simulink model "MPCController"  (R2024a)
settings: configuration reference "csMultiInstance" (kept outside this file)
undefined symbols (not defined in the file or in its folder): longVelLlimit, longVelUlimit, mioIgnoreDistanceThreshold, mioIgnoreRelDistance, mioIgnoreVelocity, time_gap, Ts
libraries: mpcadaslib x1
Description:
  | Model Predictive Controller Model. This is considered as a SW unit.
settings Model: DataDictionary=DD_MPCController.sldd  EnableAccessToBaseWorkspace=off  Creator=The MathWorks, Inc.  LastModifiedBy=The MathWorks, Inc.
settings ConfigSetRef: SourceName=csMultiInstance

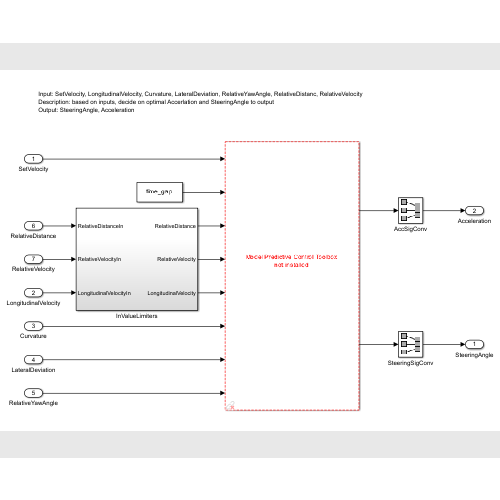
[thumbnail: Simulink's stored preview of the top-level diagram]
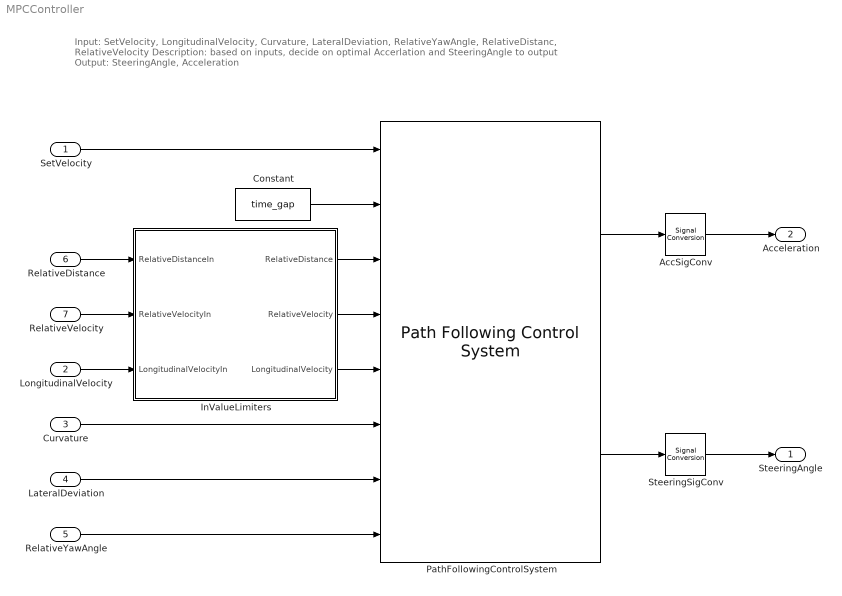
== system MPCController ==
  note: Input: SetVelocity, LongitudinalVelocity, Curvature, LateralDeviation, RelativeYawAngle, RelativeDistanc, RelativeVelocity
      | Description: based on inputs, decide on optimal Accerlation and SteeringAngle to output
      | Output: SteeringAngle, Acceleration
  SetVelocity : Inport  OutMin=-realmax  OutMax=realmax  OutDataTypeStr=double  Unit=m/s  PortDimensions=1  SampleTime=Ts
  LongitudinalVelocity : Inport  Port=2  OutMin=-realmax  OutMax=realmax  OutDataTypeStr=double  Unit=m/s  PortDimensions=1  SampleTime=Ts
  Curvature : Inport  Port=3  OutMin=-realmax  OutMax=realmax  OutDataTypeStr=double  PortDimensions=PredictionNumSteps  SampleTime=Ts
  LateralDeviation : Inport  Port=4  OutMin=-realmax  OutMax=realmax  OutDataTypeStr=double  PortDimensions=1  SampleTime=Ts
  RelativeYawAngle : Inport  Port=5  OutMin=-realmax  OutMax=realmax  OutDataTypeStr=double  Unit=rad  PortDimensions=1  SampleTime=Ts
  RelativeDistance : Inport  Port=6  OutMin=-realmax  OutMax=realmax  OutDataTypeStr=double  Unit=m  PortDimensions=1  SampleTime=Ts
  RelativeVelocity : Inport  Port=7  OutMin=-realmax  OutMax=realmax  OutDataTypeStr=double  Unit=m/s  PortDimensions=1  SampleTime=Ts
  AccSigConv : SignalConversion  OverrideOpt=off
  Constant : Constant  Value=time_gap
  InValueLimiters : Subsystem
  PathFollowingControlSystem : mpcadaslib/Path Following Control System  VariantControl=Variant2  ModelType=Use vehicle parameters  VehicleMass=m  VehicleYawInertia=Iz  LengthToFront=lf  LengthToRear=lr  FrontTireStiffness=Cf  RearTireStiffness=Cr  AccelTimeConstant=tau  EgoModelMatrixA=[-2,zeros(1,3);1,zeros(1,3);zeros(1,2),-4.4021,-12.4603;zeros(1,2),1.3913,-5.1868]  EgoModelMatrixB=[2,zeros(1,3);zeros(1,2),24.1270,15.8609]'  EgoModelMatrixC=[zeros(3,1),eye(3)]  InitialLongVel=v0_ego  TransportLag=Ts  spaceCtrl=on  DefaultSpacing=default_spacing  MinSteering=min_steer  umin_ext=off  MaxSteering=max_steer  umax_ext=off  MinAcceleration=min_ac  amin_ext=off  MaxAcceleration=max_ac  amax_ext=off  Ts=Ts  PredictionHorizon=30  ControlHorizon=3  LongWeight=0.1  LateralWeight=1  AccelRateWeight=0.1  SteerRateWeight=0.1  suboptimal=off  maxiter=10  datatypeopt=double  optmode=off  trackmode=off
  SteeringSigConv : SignalConversion  OverrideOpt=off
  SteeringAngle : Outport  OutMin=-realmax  OutMax=realmax  OutDataTypeStr=double  Unit=rad  PortDimensions=1  SampleTime=Ts  VectorParamsAs1DForOutWhenUnconnected=off
  Acceleration : Outport  Port=2  OutMin=-realmax  OutMax=realmax  OutDataTypeStr=double  Unit=m/s^2  PortDimensions=1  SampleTime=Ts  VectorParamsAs1DForOutWhenUnconnected=off
  wires:
  RelativeYawAngle/1 -> PathFollowingControlSystem/8
  PathFollowingControlSystem/1 -> AccSigConv/1
  PathFollowingControlSystem/2 -> SteeringSigConv/1
  LateralDeviation/1 -> PathFollowingControlSystem/7
  Curvature/1 -> PathFollowingControlSystem/6
  SetVelocity/1 -> PathFollowingControlSystem/1
  Constant/1 -> PathFollowingControlSystem/2
  RelativeDistance/1 -> InValueLimiters/1(RelativeDistanceIn)
  RelativeVelocity/1 -> InValueLimiters/2(RelativeVelocityIn)
  LongitudinalVelocity/1 -> InValueLimiters/3(LongitudinalVelocityIn)
  InValueLimiters/1(RelativeDistance) -> PathFollowingControlSystem/3
  InValueLimiters/2(RelativeVelocity) -> PathFollowingControlSystem/4
  InValueLimiters/3(LongitudinalVelocity) -> PathFollowingControlSystem/5
  SteeringSigConv/1 -> SteeringAngle/1
  AccSigConv/1 -> Acceleration/1

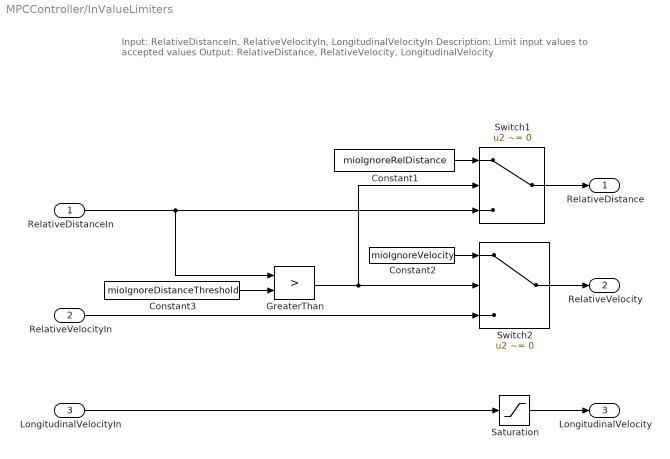
== system MPCController/InValueLimiters ==
  note: Input: RelativeDistanceIn, RelativeVelocityIn, LongitudinalVelocityIn
      | Description: Limit input values to accepted values
      | Output: RelativeDistance, RelativeVelocity, LongitudinalVelocity
  RelativeDistanceIn : Inport
  RelativeVelocityIn : Inport  Port=2
  LongitudinalVelocityIn : Inport  Port=3
  Constant1 : Constant  Value=mioIgnoreRelDistance  OutDataTypeStr=double
  Constant2 : Constant  Value=mioIgnoreVelocity  OutDataTypeStr=double
  Constant3 : Constant  Value=mioIgnoreDistanceThreshold  OutDataTypeStr=double
  GreaterThan : RelationalOperator  Operator=>  RndMeth=Simplest
  Saturation : Saturate  UpperLimit=longVelUlimit  LowerLimit=longVelLlimit
      settings: AttributesFormatString=|
      | %<LowerLimit>
      | %<UpperLimit>
  Switch1 : Switch  Criteria=u2 ~= 0  SaturateOnIntegerOverflow=off  InputSameDT=off
  Switch2 : Switch  Criteria=u2 ~= 0  SaturateOnIntegerOverflow=off  InputSameDT=off
  RelativeDistance : Outport
  RelativeVelocity : Outport  Port=2
  LongitudinalVelocity : Outport  Port=3
  wires:
  Saturation/1 -> LongitudinalVelocity/1
  Constant1/1 -> Switch1/1
  Constant2/1 -> Switch2/1
  Switch1/1 -> RelativeDistance/1
  LongitudinalVelocityIn/1 -> Saturation/1
  RelativeVelocityIn/1 -> Switch2/3
  Switch2/1 -> RelativeVelocity/1
  RelativeDistanceIn/1 -> GreaterThan/1, Switch1/3
  Constant3/1 -> GreaterThan/2
  GreaterThan/1 -> Switch1/2, Switch2/2
